simulink model "TORQUES"  (R2015a)
settings: Solver=ode45  StartTime=0.0  StopTime=10.0  RelTol=1e-3
undefined symbols (not defined in the file): Jw_fl, Jw_fr, Jw_rl, Jw_rr
settings Model: Creator=BML  LastModifiedBy=BML

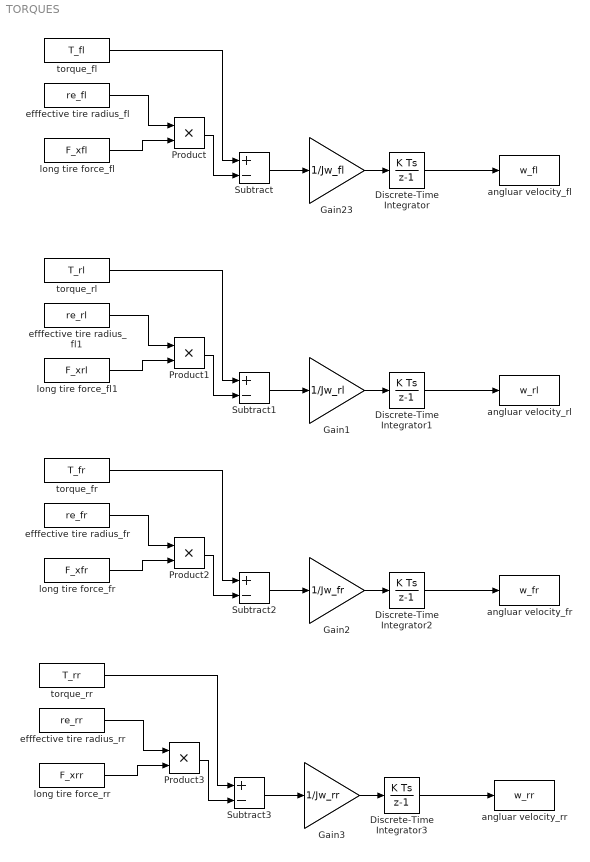
== system TORQUES ==
  Discrete-Time Integrator{,1..3} (4 alike) : DiscreteIntegrator  InitialConditionSetting=State (most efficient)
  Gain1 : Gain  Gain=1/Jw_rl
  Gain2 : Gain  Gain=1/Jw_fr
  Gain23 : Gain  Gain=1/Jw_fl
  Gain3 : Gain  Gain=1/Jw_rr
  Product{,1..3} (4 alike) : Product
  Subtract{,1..3} (4 alike) : Sum  Inputs=+-
  angluar velocity_fl : ToWorkspace  VariableName=w_fl  SaveFormat=Timeseries  SampleTime=-1
  angluar velocity_fr : ToWorkspace  VariableName=w_fr  SaveFormat=Timeseries  SampleTime=-1
  angluar velocity_rl : ToWorkspace  VariableName=w_rl  SaveFormat=Timeseries  SampleTime=-1
  angluar velocity_rr : ToWorkspace  VariableName=w_rr  SaveFormat=Timeseries  SampleTime=-1
  efffective tire radius_fl : FromWorkspace  VariableName=re_fl  SampleTime=0
  efffective tire radius_fl1 : FromWorkspace  VariableName=re_rl  SampleTime=0
  efffective tire radius_fr : FromWorkspace  VariableName=re_fr  SampleTime=0
  efffective tire radius_rr : FromWorkspace  VariableName=re_rr  SampleTime=0
  long tire force_fl : FromWorkspace  VariableName=F_xfl  SampleTime=0
  long tire force_fl1 : FromWorkspace  VariableName=F_xrl  SampleTime=0
  long tire force_fr : FromWorkspace  VariableName=F_xfr  SampleTime=0
  long tire force_rr : FromWorkspace  VariableName=F_xrr  SampleTime=0
  torque_fl : FromWorkspace  VariableName=T_fl  SampleTime=0
  torque_fr : FromWorkspace  VariableName=T_fr  SampleTime=0
  torque_rl : FromWorkspace  VariableName=T_rl  SampleTime=0
  torque_rr : FromWorkspace  VariableName=T_rr  SampleTime=0
  wires:
  efffective tire radius_fl/1 -> Product/1
  long tire force_fl/1 -> Product/2
  torque_fl/1 -> Subtract/1
  Product/1 -> Subtract/2
  Subtract/1 -> Gain23/1
  Gain23/1 -> Discrete-Time Integrator/1
  Discrete-Time Integrator/1 -> angluar velocity_fl/1
  efffective tire radius_fl1/1 -> Product1/1
  long tire force_fl1/1 -> Product1/2
  torque_rl/1 -> Subtract1/1
  Product1/1 -> Subtract1/2
  Subtract1/1 -> Gain1/1
  Gain1/1 -> Discrete-Time Integrator1/1
  Discrete-Time Integrator1/1 -> angluar velocity_rl/1
  efffective tire radius_fr/1 -> Product2/1
  long tire force_fr/1 -> Product2/2
  torque_fr/1 -> Subtract2/1
  Product2/1 -> Subtract2/2
  Subtract2/1 -> Gain2/1
  Gain2/1 -> Discrete-Time Integrator2/1
  Discrete-Time Integrator2/1 -> angluar velocity_fr/1
  efffective tire radius_rr/1 -> Product3/1
  long tire force_rr/1 -> Product3/2
  torque_rr/1 -> Subtract3/1
  Product3/1 -> Subtract3/2
  Subtract3/1 -> Gain3/1
  Gain3/1 -> Discrete-Time Integrator3/1
  Discrete-Time Integrator3/1 -> angluar velocity_rr/1
